simulink model "EV_2"  (R2023a)
settings: Solver=VariableStepAuto  StartTime=0.0  StopTime=.1  RelTol=1e-3
undefined symbols (not defined in the file or in its folder): Ion, Lithium
libraries: spsSeriesRLCBranchLib x14, spsIdealSwitchLib x10, slpidlib x9, spsMosfetLib x8, spsPWMGeneratorDCDCLib x6, spsVoltageMeasurementLib x5, spsThreePhaseVIMeasurementLib x3, spsUniversalBridgeLib x2, spsBatteryLib x1, spsThreePhaseSourceLib x1, spsThreePhaseSeriesRLCLoadLib x1, eePowerMeasurement x1
(part 2 of 2)

== matlab function EV_2/MATLAB Function1 ==
  data: t input; control output; soc input
function control = controller(t, soc)
% This function decides whether EV should charge (G2V) or discharge (V2G)
% based on electricity price (time-of-day) and battery SOC

% ---------------------------------------------------------
% STEP 1: Convert simulation time (seconds) to hour (0–24)
% ---------------------------------------------------------
hour = mod(24*t, 24);  
% Simulink time is in seconds → convert to hours
% mod(...,24) ensures it repeats every 24-hour cycle

% ---------------------------------------------------------
% STEP 2: Define SOC safety limits
% ---------------------------------------------------------
SOC_min = 59.99;  
% Minimum SOC → avoid deep discharge (battery protection)

SOC_max = 60.01;  
% Maximum SOC → avoid overcharging

% ---------------------------------------------------------
% STEP 3: Define realistic electricity price (₹/unit)
% based on time-of-day (4 slabs)
% ---------------------------------------------------------
if (hour >= 10 && hour < 16)
    price = 4;    
    % Midday (solar hours) → cheapest electricity

elseif (hour >= 16 && hour < 22)
    price = 10;   
    % Evening peak → highest demand → expensive

elseif (hour >= 6 && hour < 10)
    price = 6;    
    % Morning → moderate demand

else
    price = 5;    
    % Night → low demand → cheaper than normal
end

% ---------------------------------------------------------
% STEP 4: Initialize control (default safe mode)
% ---------------------------------------------------------
control = 0;  
% Default = 0 → charging (safe fallback)
% We avoid unnecessary discharging unless conditions are met

% ---------------------------------------------------------
% STEP 5: Decision logic (main control intelligence)
% ---------------------------------------------------------

% Case 1: High price → sell energy to grid (V2G)
if (price >= 9) && (soc > SOC_min)
    control = 1;  
    % Discharge only if:
    % - electricity is expensive
    % - battery has enough charge

% Case 2: Low price → charge battery (G2V)
elseif (price <= 5) && (soc < SOC_max)
    control = 0;  
    % Charge only if:
    % - electricity is cheap
    % - battery is not full

% Case 3: Medium price → do nothing (idle behavior)
else
    control = 0;  
    % Avoid unnecessary switching
    % keeps system stable and realistic
end

end
